simulink model "Airframe"  (R2024a)
settings: Solver=VariableStepAuto  StartTime=0.0  StopTime=10.0  RelTol=1e-3
libraries: RCTblocks x2
settings Model: Creator=Thoma  LastModifiedBy=Thoma

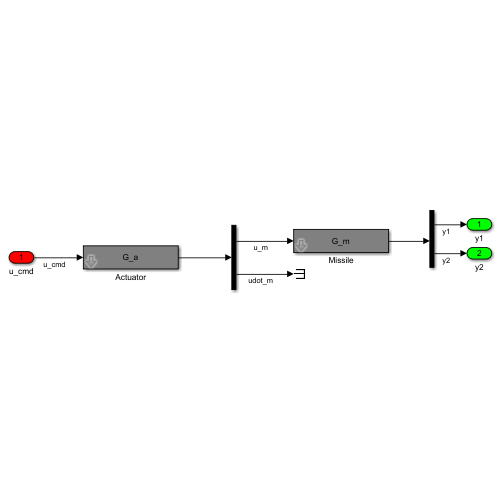
[thumbnail: Simulink's stored preview of the top-level diagram]
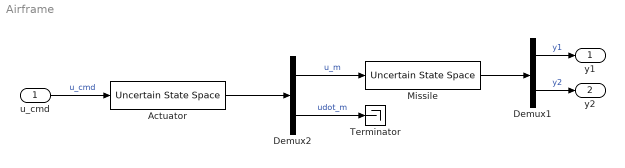
== system Airframe ==
  u_cmd : Inport
  Actuator : RCTblocks/Uncertain State Space  Tag=USS  USystem=G_a  UValue=[]  X0=[]  uX0=[]
  Demux1 : Demux  Outputs=2
  Demux2 : Demux  Outputs=2
  Missile : RCTblocks/Uncertain State Space  Tag=USS  USystem=G_m  UValue=[]  X0=[]  uX0=[]
  Terminator : Terminator
  y1 : Outport
  y2 : Outport  Port=2
  wires:
  u_cmd/1 -> Actuator/1  "u_cmd"
  Actuator/1 -> Demux2/1
  Missile/1 -> Demux1/1
  Demux1/2 -> y2/1  "y2"
  Demux1/1 -> y1/1  "y1"
  Demux2/2 -> Terminator/1  "udot_m"
  Demux2/1 -> Missile/1  "u_m"
